simulink model "quad_copter_scratch"  (R2016a)
settings: Solver=VariableStepAuto  StartTime=0.0  StopTime=30  RelTol=1e-3
undefined symbols (not defined in the file): InnerReferenceModel, Mixer, OptimalController, PitchRateModel_dt, PitchRateModel_tf, ReferenceModel_dt, Ri_tf, time_step, Ts
settings Model: Creator=tibo  LastModifiedBy=tibo

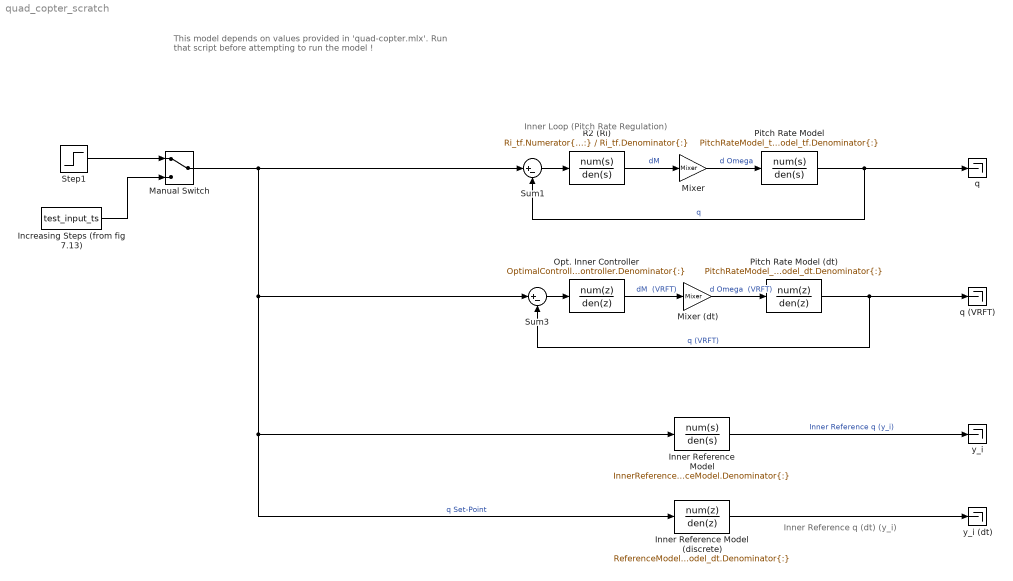
== system quad_copter_scratch ==
  note: Inner Reference q (dt) (y_i)
  note: This model depends on values provided in 'quad-copter.mlx'.
      | Run that script before attempting to run the model !
  note: Inner Loop (Pitch Rate Regulation)
  Increasing Steps (from fig 7.13) : FromWorkspace  VariableName=test_input_ts  SampleTime=time_step  OutputAfterFinalValue=Holding final value
  Inner Reference Model : TransferFcn  Numerator=InnerReferenceModel.Numerator{:}  Denominator=InnerReferenceModel.Denominator{:}
  Inner Reference Model (discrete) : DiscreteTransferFcn  Numerator=ReferenceModel_dt.Numerator{:}  Denominator=ReferenceModel_dt.Denominator{:}  SampleTime=Ts
  Manual Switch : ManualSwitch
  "Mixer " : Gain  Gain=Mixer
  Mixer (dt) : Gain  Gain=Mixer
  Opt. Inner Controller : DiscreteTransferFcn  Numerator=OptimalController.Numerator{:}  Denominator=OptimalController.Denominator{:}  SampleTime=Ts
  "Pitch Rate Model " : TransferFcn  Numerator=PitchRateModel_tf.Numerator{:}  Denominator=PitchRateModel_tf.Denominator{:}  ContinuousStateAttributes='PitchRate'
  Pitch Rate Model (dt) : DiscreteTransferFcn  Numerator=PitchRateModel_dt.Numerator{:}  Denominator=PitchRateModel_dt.Denominator{:}  SampleTime=Ts
  "R2 (Ri) " : TransferFcn  Numerator=Ri_tf.Numerator{:}  Denominator=Ri_tf.Denominator{:}
  Step1 : Step  SampleTime=0
  Sum1 : Sum  Inputs=|+-
  Sum3 : Sum  Inputs=|+-
  q : Terminator
  q (VRFT) : Terminator
  y_i : Terminator
  y_i (dt) : Terminator
  wires:
  Manual Switch/1 -> Sum1/1, Inner Reference Model (discrete)/1, Inner Reference Model/1, Sum3/1  "q Set-Point"
  "R2 (Ri) "/1 -> "Mixer "/1  "dM"
  "Mixer "/1 -> "Pitch Rate Model "/1  "d Omega"
  "Pitch Rate Model "/1 -> q/1, Sum1/2  "q"
  Increasing Steps (from fig 7.13)/1 -> Manual Switch/2
  Step1/1 -> Manual Switch/1
  Sum1/1 -> "R2 (Ri) "/1
  Opt. Inner Controller/1 -> Mixer (dt)/1  "dM  (VRFT)"
  Mixer (dt)/1 -> Pitch Rate Model (dt)/1  "d Omega  (VRFT)"
  Pitch Rate Model (dt)/1 -> q (VRFT)/1, Sum3/2  "q (VRFT)"
  Sum3/1 -> Opt. Inner Controller/1
  Inner Reference Model/1 -> y_i/1  "Inner Reference q (y_i)"
  Inner Reference Model (discrete)/1 -> y_i (dt)/1
